simulink model "znn_we3"  (R2016b)
settings: Solver=VariableStepAuto  StartTime=0.0  StopTime=512  RelTol=1e-3  EnableMultiTasking=on
undefined symbols (not defined in the file): a, b
libraries: xbsIndex_r4 x143, simulink x3
settings Model: Creator=brad  LastModifiedBy=Brad Taylor
settings OptimizationCC: LifeSpan=inf
settings DebuggingCC: SFUnexpectedBacktrackingDiag=warning  SFNoUnconditionalDefaultTransitionDiag=warning  SFExecutionAtInitializationDiag=none
settings GRTTargetCC: TargetLangStandard=C89/C90 (ANSI)  GeneratePreprocessorConditionals=Disable all
settings ConfigComp: CovMetricSettings=dw  CovHtmlReporting=on  CovSaveCumulativeToWorkspaceVar=on  CovSaveSingleToWorkspaceVar=on  CovExternalEMLEnable=off

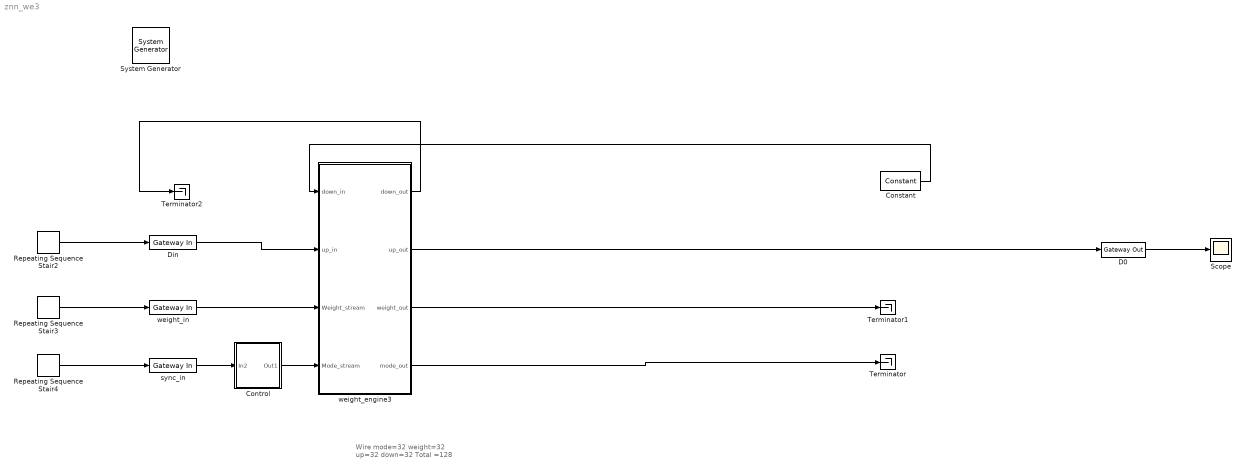
== system znn_we3 ==
  note: Wire
      | mode=32
      | weight=32
      | up=32
      | down=32
      | Total =128
  " System Generator" : xbsIndex_r4/ System Generator  Tag=genX  xilinxfamily=zynq  part=xc7z020  speed=-1  package=clg484  synthesis_tool=Vivado  clock_wrapper=Clock Enables  directory=D:/xsys/xwork/znn_we3  proj_type=Vivado  Synth_file=Vivado Synthesis Defaults  Impl_file=Vivado Implementation Defaults  testbench=off  simulink_period=1  sysclk_period=3.33  dcm_input_clock_period=10  incr_netlist=off  trim_vbits=Everywhere in SubSystem  dbl_ovrd=According to Block Masks  core_generation=According to Block Masks  run_coregen=off  deprecated_control=off  eval_field=0  block_type=sysgen
  Constant : xbsIndex_r4/Constant  const=1.0  gui_display_data_type=Fixed-point  arith_type=Unsigned  n_bits=36  bin_pt=0  preci_type=Single  exp_width=8  frac_width=24  explicit_period=on  period=1  equ=P=C  opselect=C  inp2=PCIN>>17  opr=+  inp1=P  carry=CIN  dbl_ovrd=off  block_type=constant
  Control : Subsystem
  D0 : xbsIndex_r4/Gateway Out  inherit_from_input=off  hdl_port=on  rows=1  columns=1  UseAsDAC=off  DACChannel='1'  interface=None  automatic_assignment=on  address_offset=hex2dec('00')  intf_name=''  intf_description=''  timing_constraint=None  locs_specified=off  LOCs={}  io_standard={}  block_type=gatewayout
  Din : xbsIndex_r4/Gateway In  gui_display_data_type=Fixed-point  arith_type=Unsigned  n_bits=36  bin_pt=0  preci_type=Single  exp_width=8  frac_width=24  rows=1  columns=1  quantization="Round  (unbiased: +/- Inf)"  overflow=Saturate  period=1  UseAsADC=off  ADCChannel='1'  interface=None  automatic_assignment=on  address_offset=hex2dec('00')  intf_name=''  intf_description=''  default_value=0  timing_constraint=None  locs_specified=off  LOCs={}  io_standard={}  inherit_from_input=off  hdl_port=on  dbl_ovrd=off  block_type=gatewayin
  Repeating Sequence Stair2 : simulink/Sources/Repeating Sequence Stair  OutValues=zeros(10,1)  tsamp=1  OutMin=[]  OutMax=[]  OutDataTypeStr=double  OutputDataTypeScalingMode=double  OutDataType=fixdt(0,8)  ConRadixGroup=Best Precision: Vector-wise  OutScaling=2^-12
  Repeating Sequence Stair3 : simulink/Sources/Repeating Sequence Stair  OutValues=1:10  tsamp=1  OutMin=[]  OutMax=[]  OutDataTypeStr=double  OutputDataTypeScalingMode=double  OutDataType=fixdt(0,8)  ConRadixGroup=Best Precision: Vector-wise  OutScaling=2^-12
  Repeating Sequence Stair4 : simulink/Sources/Repeating Sequence Stair  OutValues=[1, zeros(100,1)' ]  tsamp=1  OutMin=[]  OutMax=[]  OutDataTypeStr=double  OutputDataTypeScalingMode=double  OutDataType=fixdt(0,8)  ConRadixGroup=Best Precision: Vector-wise  OutScaling=2^-12
  Scope : Scope
  Terminator : Terminator
  Terminator1 : Terminator
  Terminator2 : Terminator
  sync_in : xbsIndex_r4/Gateway In  gui_display_data_type=Fixed-point  arith_type=Unsigned  n_bits=1  bin_pt=0  preci_type=Single  exp_width=8  frac_width=24  rows=1  columns=1  quantization="Round  (unbiased: +/- Inf)"  overflow=Saturate  period=1  UseAsADC=off  ADCChannel='1'  interface=None  automatic_assignment=on  address_offset=hex2dec('00')  intf_name=''  intf_description=''  default_value=0  timing_constraint=None  locs_specified=off  LOCs={}  io_standard={}  inherit_from_input=off  hdl_port=on  dbl_ovrd=off  block_type=gatewayin
  weight_engine3 : Subsystem
  weight_in : xbsIndex_r4/Gateway In  gui_display_data_type=Fixed-point  arith_type=Unsigned  n_bits=36  bin_pt=0  preci_type=Single  exp_width=8  frac_width=24  rows=1  columns=1  quantization="Round  (unbiased: +/- Inf)"  overflow=Saturate  period=1  UseAsADC=off  ADCChannel='1'  interface=None  automatic_assignment=on  address_offset=hex2dec('00')  intf_name=''  intf_description=''  default_value=0  timing_constraint=None  locs_specified=off  LOCs={}  io_standard={}  inherit_from_input=off  hdl_port=on  dbl_ovrd=off  block_type=gatewayin
  wires:
  D0/1 -> Scope/1
  Repeating Sequence Stair2/1 -> Din/1
  Repeating Sequence Stair3/1 -> weight_in/1
  Repeating Sequence Stair4/1 -> sync_in/1
  weight_engine3/3(weight_out) -> Terminator1/1
  weight_engine3/4(mode_out) -> Terminator/1
  Control/1(Out1) -> weight_engine3/4(Mode_stream)
  weight_in/1 -> weight_engine3/3(Weight_stream)
  sync_in/1 -> Control/1(In2)
  weight_engine3/2(up_out) -> D0/1
  Din/1 -> weight_engine3/2(up_in)
  weight_engine3/1(down_out) -> Terminator2/1
  Constant/1 -> weight_engine3/1(down_in)

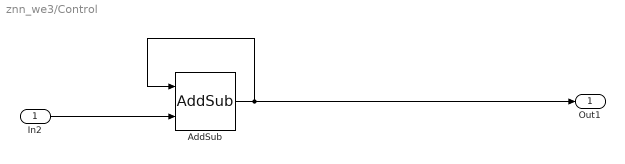
== system znn_we3/Control ==
  In2 : Inport
  AddSub : xbsIndex_r4/AddSub  mode=Addition  use_carryin=off  use_carryout=off  en=off  latency=1  precision=User Defined  arith_type=Unsigned  n_bits=36  bin_pt=0  quantization=Truncate  overflow=Wrap  use_behavioral_HDL=off  hw_selection=Fabric  pipelined=off  dbl_ovrd=off  block_type=addsub
  Out1 : Outport
  wires:
  In2/1 -> AddSub/2
  AddSub/1 -> AddSub/1, Out1/1

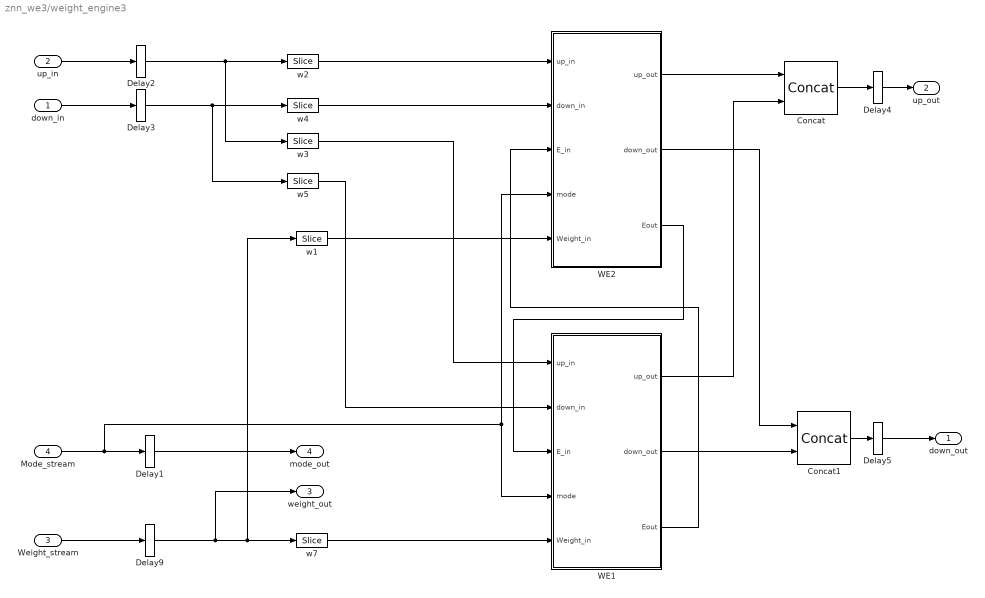
== system znn_we3/weight_engine3 ==
  down_in : Inport
  up_in : Inport  Port=2
  Weight_stream : Inport  Port=3
  Mode_stream : Inport  Port=4
  Concat : xbsIndex_r4/Concat  num_inputs=2  dbl_ovrd=off  block_type=concat
  Concat1 : xbsIndex_r4/Concat  num_inputs=2  dbl_ovrd=off  block_type=concat
  Delay{1..5,9} (6 alike) : xbsIndex_r4/Delay  rst=off  infoeditControl=Selection of Reset will increase slice count due to use of real FFs and instead of SRLs  en=off  latency=1  reg_retiming=off  dbl_ovrd=off  block_type=delay
      settings: infoedit=Hardware notes: A delay line is a chain, each link of which is an SRL16 or SRL32 followed by a flip-flop.
  WE1 : Subsystem
  WE2 : Subsystem
  w1 : xbsIndex_r4/Slice  nbits=1  boolean_output=off  mode=Two Bit Locations  bit1=35  base1=LSB of Input  bit0=18  base0=LSB of Input  dbl_ovrd=off  block_type=slice
  w2 : xbsIndex_r4/Slice  nbits=1  boolean_output=off  mode=Two Bit Locations  bit1=35  base1=LSB of Input  bit0=18  base0=LSB of Input  dbl_ovrd=off  block_type=slice
  w3 : xbsIndex_r4/Slice  nbits=1  boolean_output=off  mode=Two Bit Locations  bit1=17  base1=LSB of Input  bit0=0  base0=LSB of Input  dbl_ovrd=off  block_type=slice
  w4 : xbsIndex_r4/Slice  nbits=1  boolean_output=off  mode=Two Bit Locations  bit1=35  base1=LSB of Input  bit0=18  base0=LSB of Input  dbl_ovrd=off  block_type=slice
  w5 : xbsIndex_r4/Slice  nbits=1  boolean_output=off  mode=Two Bit Locations  bit1=17  base1=LSB of Input  bit0=0  base0=LSB of Input  dbl_ovrd=off  block_type=slice
  w7 : xbsIndex_r4/Slice  nbits=1  boolean_output=off  mode=Two Bit Locations  bit1=17  base1=LSB of Input  bit0=0  base0=LSB of Input  dbl_ovrd=off  block_type=slice
  down_out : Outport
  up_out : Outport  Port=2
  weight_out : Outport  Port=3
  mode_out : Outport  Port=4
  wires:
  Weight_stream/1 -> Delay9/1
  Delay9/1 -> weight_out/1, w7/1, w1/1
  WE2/2(down_out) -> Concat1/1
  down_in/1 -> Delay3/1
  Mode_stream/1 -> Delay1/1, WE2/4(mode), WE1/4(mode)
  WE1/2(down_out) -> Concat1/2
  WE1/1(up_out) -> Concat/2
  WE1/3(Eout) -> WE2/3(E_in)
  WE2/3(Eout) -> WE1/3(E_in)
  w7/1 -> WE1/5(Weight_in)
  w1/1 -> WE2/5(Weight_in)
  Concat/1 -> Delay4/1
  Concat1/1 -> Delay5/1
  w2/1 -> WE2/1(up_in)
  up_in/1 -> Delay2/1
  w3/1 -> WE1/1(up_in)
  w4/1 -> WE2/2(down_in)
  w5/1 -> WE1/2(down_in)
  Delay1/1 -> mode_out/1
  Delay2/1 -> w3/1, w2/1
  Delay3/1 -> w5/1, w4/1
  Delay4/1 -> up_out/1
  Delay5/1 -> down_out/1
  WE2/1(up_out) -> Concat/1

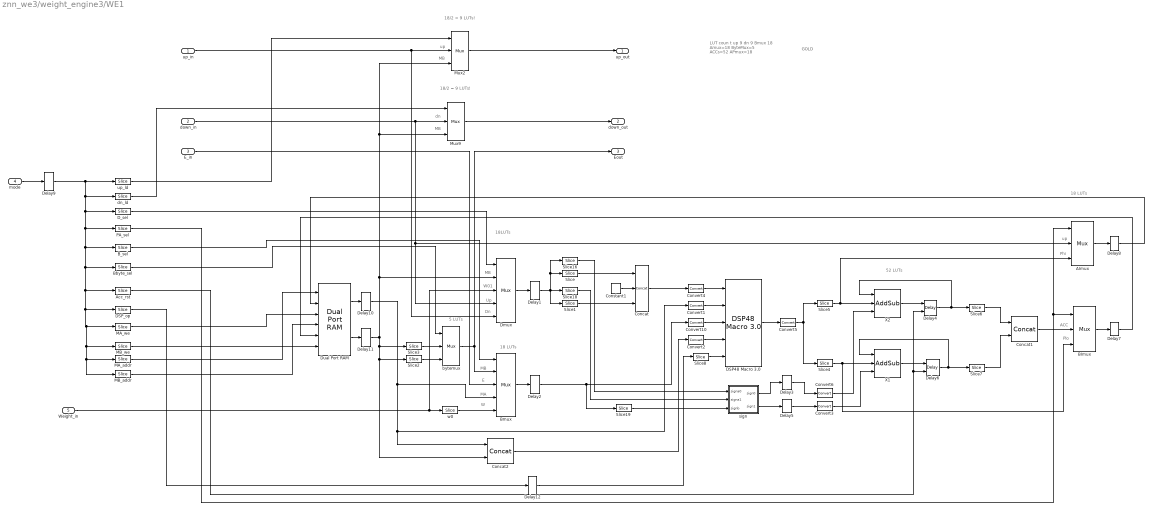
== system znn_we3/weight_engine3/WE1 ==
  note: Plo
  note: ACC
  note: Phi
  note: up
  note: MB
  note: dn
  note: MB
  note: up
  note: 5 LUTs
  note: Dn
  note: Up
  note: W01
  note: MB
  note: W
  note: E
  note: GOLD
  note: LUT coun t
      | up 9
      | dn 9
      | Bmux 18
      | Amux=18
      | ByteMux=5
      | ACCs=52
      | APmux=18
  note: 18 LUTs
  note: 18LUTs
  note: 18 LUTs
  note: 52 LUTs
  note: MA
  note: MB
  note: 18/2 = 9 LUTs!
  note: 18/2 = 9 LUTs!
  up_in : Inport
  down_in : Inport  Port=2
  E_in : Inport  Port=3
  mode : Inport  Port=4
  Weight_in : Inport  Port=5
  AImux : xbsIndex_r4/Mux  inputs=2  en=off  latency=0  precision=Full  arith_type=Unsigned  n_bits=16  bin_pt=14  quantization=Truncate  overflow=Wrap  dbl_ovrd=off  block_type=mux
  Acc_rst : xbsIndex_r4/Slice  nbits=1  boolean_output=on  mode=Two Bit Locations  bit1=26  base1=LSB of Input  bit0=26  base0=LSB of Input  dbl_ovrd=off  block_type=slice
  BImux : xbsIndex_r4/Mux  inputs=2  en=off  latency=0  precision=Full  arith_type=Unsigned  n_bits=16  bin_pt=14  quantization=Truncate  overflow=Wrap  dbl_ovrd=off  block_type=mux
  B_sel : xbsIndex_r4/Slice  nbits=1  boolean_output=off  mode=Two Bit Locations  bit1=29  base1=LSB of Input  bit0=28  base0=LSB of Input  dbl_ovrd=off  block_type=slice
  Bbyte_sel : xbsIndex_r4/Slice  nbits=1  boolean_output=off  mode=Two Bit Locations  bit1=27  base1=LSB of Input  bit0=27  base0=LSB of Input  dbl_ovrd=off  block_type=slice
  Bmux : xbsIndex_r4/Mux  inputs=4  en=off  latency=0  precision=Full  arith_type=Unsigned  n_bits=16  bin_pt=14  quantization=Truncate  overflow=Wrap  dbl_ovrd=off  block_type=mux
  Concat : xbsIndex_r4/Concat  num_inputs=3  dbl_ovrd=off  block_type=concat
  Concat1 : xbsIndex_r4/Concat  num_inputs=2  dbl_ovrd=off  block_type=concat
  Concat2 : xbsIndex_r4/Concat  num_inputs=2  dbl_ovrd=off  block_type=concat
  Constant1 : xbsIndex_r4/Constant  const=0  gui_display_data_type=Fixed-point  arith_type=Unsigned  n_bits=8  bin_pt=0  preci_type=Single  exp_width=8  frac_width=24  explicit_period=off  period=1  equ=P=C  opselect=C  inp2=PCIN>>17  opr=+  inp1=P  carry=CIN  dbl_ovrd=off  block_type=constant
  Convert1 : xbsIndex_r4/Convert  gui_display_data_type=Fixed-point  arith_type="Signed  (2's comp)"  n_bits=18  bin_pt=0  float_type=Single  exp_bits=8  fraction_bits=24  quantization=Truncate  overflow=Wrap  en=off  latency=0  pipeline=off  dbl_ovrd=off  block_type=convert
  Convert10 : xbsIndex_r4/Convert  gui_display_data_type=Fixed-point  arith_type="Signed  (2's comp)"  n_bits=18  bin_pt=0  float_type=Single  exp_bits=8  fraction_bits=24  quantization=Truncate  overflow=Wrap  en=off  latency=0  pipeline=off  dbl_ovrd=off  block_type=convert
  Convert2 : xbsIndex_r4/Convert  gui_display_data_type=Fixed-point  arith_type="Signed  (2's comp)"  n_bits=36  bin_pt=0  float_type=Single  exp_bits=8  fraction_bits=24  quantization=Truncate  overflow=Wrap  en=off  latency=0  pipeline=off  dbl_ovrd=off  block_type=convert
  Convert3 : xbsIndex_r4/Convert  gui_display_data_type=Boolean  arith_type=Boolean  n_bits=9  bin_pt=0  float_type=Single  exp_bits=8  fraction_bits=24  quantization=Truncate  overflow=Wrap  en=off  latency=0  pipeline=off  dbl_ovrd=off  block_type=convert
  Convert4 : xbsIndex_r4/Convert  gui_display_data_type=Fixed-point  arith_type="Signed  (2's comp)"  n_bits=23  bin_pt=0  float_type=Single  exp_bits=8  fraction_bits=24  quantization=Truncate  overflow=Wrap  en=off  latency=0  pipeline=off  dbl_ovrd=off  block_type=convert
  Convert5 : xbsIndex_r4/Convert  gui_display_data_type=Fixed-point  arith_type=Unsigned  n_bits=48  bin_pt=0  float_type=Single  exp_bits=8  fraction_bits=24  quantization=Truncate  overflow=Wrap  en=off  latency=0  pipeline=off  dbl_ovrd=off  block_type=convert
  Convert6 : xbsIndex_r4/Convert  gui_display_data_type=Boolean  arith_type=Boolean  n_bits=9  bin_pt=0  float_type=Single  exp_bits=8  fraction_bits=24  quantization=Truncate  overflow=Wrap  en=off  latency=0  pipeline=off  dbl_ovrd=off  block_type=convert
  "DSP48 Macro 3.0 " : xbsIndex_r4/DSP48 Macro 3.0   dsptype=Target XtremeDSP Slice: DSP48E1  instruction_list=|  show_filtered=on  pipeline_options=By_Tier  dspimage=?  tier_1=off  tier_2=off  tier_3=off  tier_4=on  tier_5=on  tier_6=on  dreg_1=off  dreg_2=off  dreg_3=off  areg_1=off  areg_2=off  areg_3=off  areg_4=on  breg_1=off  breg_2=off  breg_3=off  breg_4=on  mreg_5=on  concatreg_3=off  concatreg_4=off  concatreg_5=off  creg_1=off  creg_2=off  creg_3=off  creg_4=on  creg_5=on  preg_6=on  cinreg_1=off  cinreg_2=off  cinreg_3=off  cinreg_4=off  cinreg_5=off  opreg_1=off  opreg_2=off  opreg_3=off  opreg_4=on  opreg_5=on  output_properties=Full_Precision  p_width=48  p_binarywidth=0  has_acout=off  has_bcout=off  has_pcout=off  has_carryout=off  has_carrycascout=off  has_ce=off  has_d_ce=off  has_a_ce=off  has_b_ce=off  has_concat_ce=off  has_c_ce=off  has_m_ce=off  has_p_ce=off  has_sel_ce=off  has_sclr=off  has_d_sclr=off  has_a_sclr=off  has_b_sclr=off  has_concat_sclr=off  has_c_sclr=off  has_m_sclr=off  has_p_sclr=off  has_sel_sclr=off  use_dsp48=on  simulation_type=fast_sim  simulation_model=sysgen:xbip_dsp48_macro_v3_0  gui_behaviour=Sysgen  instruction1='#'  ip_name=DSP48 Macro  ip_version=3.0  dsptool_ready=true  ipcore_usecache=true  ipcore_useipmodelcache=true  wrapper_available=true  port_translation_map={ 'ce' => 'en', 'sclr' => 'rst'}  ipcore_latency_function='has_combinational'  structural_sim=false  ipcore_verbose=false  ipcore_port_config={ 'carryin' => { 'arith' => 'ufix', 'binpt' => 0.00000000000, 'width' => 1.00000000000}, 'carrycascin' => { 'arith' => 'ufix', 'binpt' => 0.00000000000, 'width' => 1.00000000000}, 'carrycascout' => { 'arith' => 'ufix', 'binpt' => 0.00000000000, 'width' => 1.00000000000}, 'carryout' => { 'arith' => 'ufix', 'binpt' => 0.00000000000, 'width' => 1.00000000000}}  ipcore_xco_need_fpga_part=true  block_type=xbip_dsp48_macro_v3_0
      | A*B
      | D*B
      | C
      settings: infoedit=<html>Valid operands: CONCAT, P, C, PCIN, P>>17, PCIN>>17, CARRYIN, CARRYCASCIN, ACIN, A, BCIN,B<br><br>Valid operators: +, -, *, ()<br><br>Valid functions: RNDSIMPLE, RNDSYM<br><br>Instructions are case insensitive and tolerate spaces.</html>
  DSP_op : xbsIndex_r4/Slice  nbits=1  boolean_output=off  mode=Two Bit Locations  bit1=25  base1=LSB of Input  bit0=22  base0=LSB of Input  dbl_ovrd=off  block_type=slice
  D_sel : xbsIndex_r4/Slice  nbits=1  boolean_output=off  mode=Two Bit Locations  bit1=32  base1=LSB of Input  bit0=31  base0=LSB of Input  dbl_ovrd=off  block_type=slice
  Delay{1..2,7..12} (8 alike) : xbsIndex_r4/Delay  rst=off  infoeditControl=Selection of Reset will increase slice count due to use of real FFs and instead of SRLs  en=off  latency=1  reg_retiming=off  dbl_ovrd=off  block_type=delay
  Delay3 : xbsIndex_r4/Delay  rst=off  infoeditControl=Selection of Reset will increase slice count due to use of real FFs and instead of SRLs  en=off  latency=3  reg_retiming=off  dbl_ovrd=off  block_type=delay
  Delay4 : xbsIndex_r4/Delay  rst=on  infoeditControl=Selection of Reset will increase slice count due to use of real FFs and instead of SRLs  en=off  latency=1  reg_retiming=off  dbl_ovrd=off  block_type=delay
  Delay5 : xbsIndex_r4/Delay  rst=off  infoeditControl=Selection of Reset will increase slice count due to use of real FFs and instead of SRLs  en=off  latency=3  reg_retiming=off  dbl_ovrd=off  block_type=delay
  Delay6 : xbsIndex_r4/Delay  rst=on  infoeditControl=Selection of Reset will increase slice count due to use of real FFs and instead of SRLs  en=off  latency=1  reg_retiming=off  dbl_ovrd=off  block_type=delay
  Dmux : xbsIndex_r4/Mux  inputs=4  en=off  latency=0  precision=Full  arith_type=Unsigned  n_bits=16  bin_pt=14  quantization=Truncate  overflow=Wrap  dbl_ovrd=off  block_type=mux
  Dual Port RAM : xbsIndex_r4/Dual Port RAM  depth=1024  initVector=1:100  distributed_mem=Block RAM  init_a=0  init_b=0  rst_a=off  rst_b=off  en_a=off  en_b=off  latency=2  write_mode_A=Read After Write  write_mode_B=Read After Write  optimize=Speed  dbl_ovrd=off  block_type=dpram
  MA_addr : xbsIndex_r4/Slice  nbits=1  boolean_output=off  mode=Two Bit Locations  bit1=19  base1=LSB of Input  bit0=10  base0=LSB of Input  dbl_ovrd=off  block_type=slice
  MA_we : xbsIndex_r4/Slice  nbits=1  boolean_output=on  mode=Two Bit Locations  bit1=21  base1=LSB of Input  bit0=21  base0=LSB of Input  dbl_ovrd=off  block_type=slice
  MB_addr : xbsIndex_r4/Slice  nbits=1  boolean_output=off  mode=Two Bit Locations  bit1=9  base1=LSB of Input  bit0=0  base0=LSB of Input  dbl_ovrd=off  block_type=slice
  MB_we : xbsIndex_r4/Slice  nbits=1  boolean_output=on  mode=Two Bit Locations  bit1=20  base1=LSB of Input  bit0=20  base0=LSB of Input  dbl_ovrd=off  block_type=slice
  Mux2 : xbsIndex_r4/Mux  inputs=2  en=off  latency=0  precision=Full  arith_type=Unsigned  n_bits=16  bin_pt=14  quantization=Truncate  overflow=Wrap  dbl_ovrd=off  block_type=mux
  Mux9 : xbsIndex_r4/Mux  inputs=2  en=off  latency=0  precision=Full  arith_type=Unsigned  n_bits=16  bin_pt=14  quantization=Truncate  overflow=Wrap  dbl_ovrd=off  block_type=mux
  PA_sel : xbsIndex_r4/Slice  nbits=1  boolean_output=off  mode=Two Bit Locations  bit1=30  base1=LSB of Input  bit0=30  base0=LSB of Input  dbl_ovrd=off  block_type=slice
  Slice : xbsIndex_r4/Slice  nbits=1  boolean_output=off  mode=Two Bit Locations  bit1=16  base1=LSB of Input  bit0=9  base0=LSB of Input  dbl_ovrd=off  block_type=slice
  Slice1 : xbsIndex_r4/Slice  nbits=1  boolean_output=off  mode=Two Bit Locations  bit1=7  base1=LSB of Input  bit0=0  base0=LSB of Input  dbl_ovrd=off  block_type=slice
  Slice16 : xbsIndex_r4/Slice  nbits=1  boolean_output=off  mode=Two Bit Locations  bit1=16  base1=LSB of Input  bit0=16  base0=LSB of Input  dbl_ovrd=off  block_type=slice
  Slice18 : xbsIndex_r4/Slice  nbits=1  boolean_output=off  mode=Two Bit Locations  bit1=8  base1=LSB of Input  bit0=8  base0=LSB of Input  dbl_ovrd=off  block_type=slice
  Slice19 : xbsIndex_r4/Slice  nbits=1  boolean_output=off  mode=Two Bit Locations  bit1=8  base1=LSB of Input  bit0=8  base0=LSB of Input  dbl_ovrd=off  block_type=slice
  Slice2 : xbsIndex_r4/Slice  nbits=1  boolean_output=off  mode=Two Bit Locations  bit1=17  base1=LSB of Input  bit0=9  base0=LSB of Input  dbl_ovrd=off  block_type=slice
  Slice3 : xbsIndex_r4/Slice  nbits=1  boolean_output=off  mode=Two Bit Locations  bit1=8  base1=LSB of Input  bit0=0  base0=LSB of Input  dbl_ovrd=off  block_type=slice
  Slice4 : xbsIndex_r4/Slice  nbits=1  boolean_output=off  mode=Two Bit Locations  bit1=17  base1=LSB of Input  bit0=0  base0=LSB of Input  dbl_ovrd=off  block_type=slice
  Slice5 : xbsIndex_r4/Slice  nbits=1  boolean_output=off  mode=Two Bit Locations  bit1=35  base1=LSB of Input  bit0=18  base0=LSB of Input  dbl_ovrd=off  block_type=slice
  Slice6 : xbsIndex_r4/Slice  nbits=1  boolean_output=off  mode=Two Bit Locations  bit1=24  base1=LSB of Input  bit0=17  base0=LSB of Input  dbl_ovrd=off  block_type=slice
  Slice7 : xbsIndex_r4/Slice  nbits=1  boolean_output=off  mode=Two Bit Locations  bit1=24  base1=LSB of Input  bit0=17  base0=LSB of Input  dbl_ovrd=off  block_type=slice
  Slice8 : xbsIndex_r4/Slice  nbits=1  boolean_output=off  mode=Two Bit Locations  bit1=1  base1=LSB of Input  bit0=0  base0=LSB of Input  dbl_ovrd=off  block_type=slice
  X1 : xbsIndex_r4/AddSub  mode=Addition or Subtraction  use_carryin=off  use_carryout=off  en=off  latency=0  precision=User Defined  arith_type="Signed  (2's comp)"  n_bits=26  bin_pt=0  quantization=Truncate  overflow=Wrap  use_behavioral_HDL=off  hw_selection=Fabric  pipelined=off  dbl_ovrd=off  block_type=addsub
  X2 : xbsIndex_r4/AddSub  mode=Addition or Subtraction  use_carryin=off  use_carryout=off  en=off  latency=0  precision=User Defined  arith_type="Signed  (2's comp)"  n_bits=26  bin_pt=0  quantization=Truncate  overflow=Wrap  use_behavioral_HDL=off  hw_selection=Fabric  pipelined=off  dbl_ovrd=off  block_type=addsub
  bytemux : xbsIndex_r4/Mux  inputs=2  en=off  latency=0  precision=Full  arith_type=Unsigned  n_bits=16  bin_pt=14  quantization=Truncate  overflow=Wrap  dbl_ovrd=off  block_type=mux
  dn_ld : xbsIndex_r4/Slice  nbits=1  boolean_output=off  mode=Two Bit Locations  bit1=33  base1=LSB of Input  bit0=33  base0=LSB of Input  dbl_ovrd=off  block_type=slice
  sign : Subsystem
  up_ld : xbsIndex_r4/Slice  nbits=1  boolean_output=off  mode=Two Bit Locations  bit1=34  base1=LSB of Input  bit0=34  base0=LSB of Input  dbl_ovrd=off  block_type=slice
  w0 : xbsIndex_r4/Slice  nbits=1  boolean_output=off  mode=Two Bit Locations  bit1=8  base1=LSB of Input  bit0=0  base0=LSB of Input  dbl_ovrd=off  block_type=slice
  up_out : Outport
  down_out : Outport  Port=2
  Eout : Outport  Port=3
  wires:
  Convert4/1 -> "DSP48 Macro 3.0 "/1
  sign/2(sign1) -> Delay5/1
  w0/1 -> Bmux/5
  Convert10/1 -> "DSP48 Macro 3.0 "/3
  Dmux/1 -> Delay1/1
  Convert1/1 -> "DSP48 Macro 3.0 "/2
  Dual Port RAM/1 -> Delay10/1
  Slice2/1 -> bytemux/3
  Slice18/1 -> sign/2(signa1)
  Slice19/1 -> sign/3(signb)
  sign/1(sign0) -> Delay3/1
  PA_sel/1 -> BImux/1, AImux/1
  B_sel/1 -> Bmux/1
  Bbyte_sel/1 -> bytemux/1
  X1/1 -> Delay6/1
  MA_addr/1 -> Dual Port RAM/1
  MA_we/1 -> Dual Port RAM/3
  Slice5/1 -> AImux/3, X2/2
  Concat1/1 -> BImux/2
  Delay6/1 -> Slice7/1, X1/1
  Convert5/1 -> Slice5/1, Slice4/1
  X2/1 -> Delay4/1
  Acc_rst/1 -> Delay4/2, Delay6/2
  Delay4/1 -> Slice6/1, X2/1
  Slice4/1 -> BImux/3, X1/2
  Convert3/1 -> X1/3
  Constant1/1 -> Concat/2
  Slice6/1 -> Concat1/1
  "DSP48 Macro 3.0 "/1 -> Convert5/1
  Slice7/1 -> Concat1/2
  BImux/1 -> Delay7/1
  MB_we/1 -> Dual Port RAM/6
  Slice1/1 -> Concat/3
  Slice/1 -> Concat/1
  Slice3/1 -> bytemux/2
  Bmux/1 -> Delay2/1
  bytemux/1 -> Eout/1, Bmux/2
  Dual Port RAM/2 -> Delay11/1
  Weight_in/1 -> Dmux/3, w0/1
  Slice16/1 -> sign/1(signa0)
  Mux9/1 -> down_out/1
  dn_ld/1 -> Mux9/1
  D_sel/1 -> Dmux/1
  down_in/1 -> AImux/2, Dmux/4, Mux9/2
  Concat2/1 -> Convert2/1
  mode/1 -> Delay9/1
  up_in/1 -> Mux2/2, Dmux/5
  MB_addr/1 -> Dual Port RAM/4
  E_in/1 -> Bmux/3
  up_ld/1 -> Mux2/1
  Convert2/1 -> "DSP48 Macro 3.0 "/4
  Convert6/1 -> X2/3
  AImux/1 -> Delay8/1
  Mux2/1 -> up_out/1
  Delay1/1 -> Slice1/1, Slice18/1, Slice/1, Slice16/1
  Delay2/1 -> Slice19/1, Convert10/1
  Delay3/1 -> Convert6/1
  Delay5/1 -> Convert3/1
  Delay7/1 -> Dual Port RAM/5
  Delay8/1 -> Dual Port RAM/2
  Concat/1 -> Convert4/1
  Slice8/1 -> "DSP48 Macro 3.0 "/5
  DSP_op/1 -> Delay12/1
  Delay9/1 -> dn_ld/1, PA_sel/1, B_sel/1, MB_addr/1, MA_addr/1, MB_we/1, MA_we/1, DSP_op/1, Acc_rst/1, Bbyte_sel/1, D_sel/1, up_ld/1
  Delay10/1 -> Bmux/4, Convert1/1, Concat2/1
  Delay11/1 -> Slice3/1, Slice2/1, Concat2/2, Mux2/3, Mux9/3, Dmux/2
  Delay12/1 -> Slice8/1

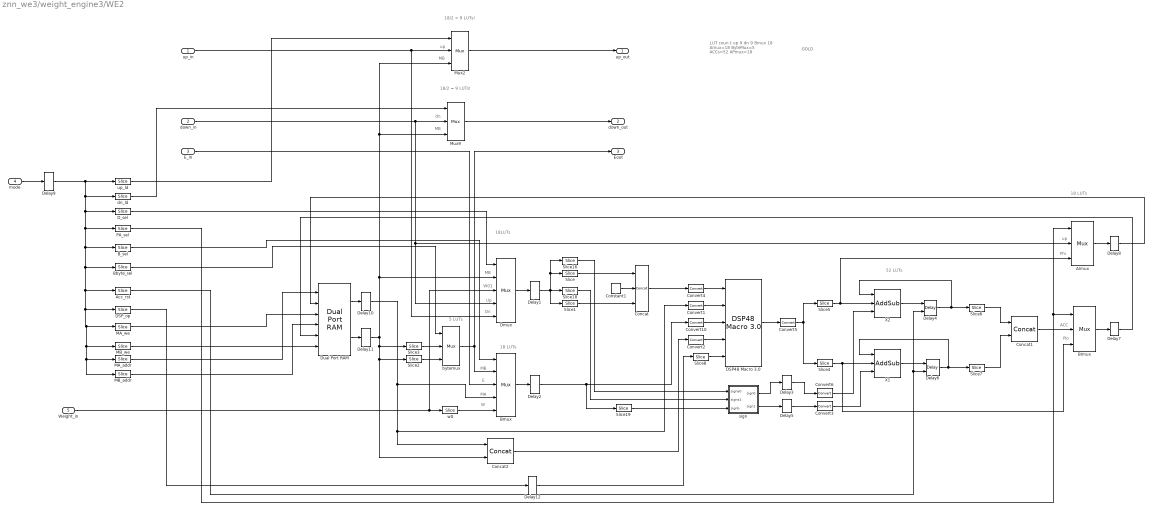
== system znn_we3/weight_engine3/WE2 ==
  note: Plo
  note: ACC
  note: Phi
  note: up
  note: MB
  note: dn
  note: MB
  note: up
  note: 5 LUTs
  note: Dn
  note: Up
  note: W01
  note: MB
  note: W
  note: E
  note: GOLD
  note: LUT coun t
      | up 9
      | dn 9
      | Bmux 18
      | Amux=18
      | ByteMux=5
      | ACCs=52
      | APmux=18
  note: 18 LUTs
  note: 18LUTs
  note: 18 LUTs
  note: 52 LUTs
  note: MA
  note: MB
  note: 18/2 = 9 LUTs!
  note: 18/2 = 9 LUTs!
  up_in : Inport
  down_in : Inport  Port=2
  E_in : Inport  Port=3
  mode : Inport  Port=4
  Weight_in : Inport  Port=5
  AImux : xbsIndex_r4/Mux  inputs=2  en=off  latency=0  precision=Full  arith_type=Unsigned  n_bits=16  bin_pt=14  quantization=Truncate  overflow=Wrap  dbl_ovrd=off  block_type=mux
  Acc_rst : xbsIndex_r4/Slice  nbits=1  boolean_output=on  mode=Two Bit Locations  bit1=26  base1=LSB of Input  bit0=26  base0=LSB of Input  dbl_ovrd=off  block_type=slice
  BImux : xbsIndex_r4/Mux  inputs=2  en=off  latency=0  precision=Full  arith_type=Unsigned  n_bits=16  bin_pt=14  quantization=Truncate  overflow=Wrap  dbl_ovrd=off  block_type=mux
  B_sel : xbsIndex_r4/Slice  nbits=1  boolean_output=off  mode=Two Bit Locations  bit1=29  base1=LSB of Input  bit0=28  base0=LSB of Input  dbl_ovrd=off  block_type=slice
  Bbyte_sel : xbsIndex_r4/Slice  nbits=1  boolean_output=off  mode=Two Bit Locations  bit1=27  base1=LSB of Input  bit0=27  base0=LSB of Input  dbl_ovrd=off  block_type=slice
  Bmux : xbsIndex_r4/Mux  inputs=4  en=off  latency=0  precision=Full  arith_type=Unsigned  n_bits=16  bin_pt=14  quantization=Truncate  overflow=Wrap  dbl_ovrd=off  block_type=mux
  Concat : xbsIndex_r4/Concat  num_inputs=3  dbl_ovrd=off  block_type=concat
  Concat1 : xbsIndex_r4/Concat  num_inputs=2  dbl_ovrd=off  block_type=concat
  Concat2 : xbsIndex_r4/Concat  num_inputs=2  dbl_ovrd=off  block_type=concat
  Constant1 : xbsIndex_r4/Constant  const=0  gui_display_data_type=Fixed-point  arith_type=Unsigned  n_bits=8  bin_pt=0  preci_type=Single  exp_width=8  frac_width=24  explicit_period=off  period=1  equ=P=C  opselect=C  inp2=PCIN>>17  opr=+  inp1=P  carry=CIN  dbl_ovrd=off  block_type=constant
  Convert1 : xbsIndex_r4/Convert  gui_display_data_type=Fixed-point  arith_type="Signed  (2's comp)"  n_bits=18  bin_pt=0  float_type=Single  exp_bits=8  fraction_bits=24  quantization=Truncate  overflow=Wrap  en=off  latency=0  pipeline=off  dbl_ovrd=off  block_type=convert
  Convert10 : xbsIndex_r4/Convert  gui_display_data_type=Fixed-point  arith_type="Signed  (2's comp)"  n_bits=18  bin_pt=0  float_type=Single  exp_bits=8  fraction_bits=24  quantization=Truncate  overflow=Wrap  en=off  latency=0  pipeline=off  dbl_ovrd=off  block_type=convert
  Convert2 : xbsIndex_r4/Convert  gui_display_data_type=Fixed-point  arith_type="Signed  (2's comp)"  n_bits=36  bin_pt=0  float_type=Single  exp_bits=8  fraction_bits=24  quantization=Truncate  overflow=Wrap  en=off  latency=0  pipeline=off  dbl_ovrd=off  block_type=convert
  Convert3 : xbsIndex_r4/Convert  gui_display_data_type=Boolean  arith_type=Boolean  n_bits=9  bin_pt=0  float_type=Single  exp_bits=8  fraction_bits=24  quantization=Truncate  overflow=Wrap  en=off  latency=0  pipeline=off  dbl_ovrd=off  block_type=convert
  Convert4 : xbsIndex_r4/Convert  gui_display_data_type=Fixed-point  arith_type="Signed  (2's comp)"  n_bits=23  bin_pt=0  float_type=Single  exp_bits=8  fraction_bits=24  quantization=Truncate  overflow=Wrap  en=off  latency=0  pipeline=off  dbl_ovrd=off  block_type=convert
  Convert5 : xbsIndex_r4/Convert  gui_display_data_type=Fixed-point  arith_type=Unsigned  n_bits=48  bin_pt=0  float_type=Single  exp_bits=8  fraction_bits=24  quantization=Truncate  overflow=Wrap  en=off  latency=0  pipeline=off  dbl_ovrd=off  block_type=convert
  Convert6 : xbsIndex_r4/Convert  gui_display_data_type=Boolean  arith_type=Boolean  n_bits=9  bin_pt=0  float_type=Single  exp_bits=8  fraction_bits=24  quantization=Truncate  overflow=Wrap  en=off  latency=0  pipeline=off  dbl_ovrd=off  block_type=convert
  "DSP48 Macro 3.0 " : xbsIndex_r4/DSP48 Macro 3.0   dsptype=Target XtremeDSP Slice: DSP48E1  instruction_list=|  show_filtered=on  pipeline_options=By_Tier  dspimage=?  tier_1=off  tier_2=off  tier_3=off  tier_4=on  tier_5=on  tier_6=on  dreg_1=off  dreg_2=off  dreg_3=off  areg_1=off  areg_2=off  areg_3=off  areg_4=on  breg_1=off  breg_2=off  breg_3=off  breg_4=on  mreg_5=on  concatreg_3=off  concatreg_4=off  concatreg_5=off  creg_1=off  creg_2=off  creg_3=off  creg_4=on  creg_5=on  preg_6=on  cinreg_1=off  cinreg_2=off  cinreg_3=off  cinreg_4=off  cinreg_5=off  opreg_1=off  opreg_2=off  opreg_3=off  opreg_4=on  opreg_5=on  output_properties=Full_Precision  p_width=48  p_binarywidth=0  has_acout=off  has_bcout=off  has_pcout=off  has_carryout=off  has_carrycascout=off  has_ce=off  has_d_ce=off  has_a_ce=off  has_b_ce=off  has_concat_ce=off  has_c_ce=off  has_m_ce=off  has_p_ce=off  has_sel_ce=off  has_sclr=off  has_d_sclr=off  has_a_sclr=off  has_b_sclr=off  has_concat_sclr=off  has_c_sclr=off  has_m_sclr=off  has_p_sclr=off  has_sel_sclr=off  use_dsp48=on  simulation_type=fast_sim  simulation_model=sysgen:xbip_dsp48_macro_v3_0  gui_behaviour=Sysgen  instruction1='#'  ip_name=DSP48 Macro  ip_version=3.0  dsptool_ready=true  ipcore_usecache=true  ipcore_useipmodelcache=true  wrapper_available=true  port_translation_map={ 'ce' => 'en', 'sclr' => 'rst'}  ipcore_latency_function='has_combinational'  structural_sim=false  ipcore_verbose=false  ipcore_port_config={ 'carryin' => { 'arith' => 'ufix', 'binpt' => 0.00000000000, 'width' => 1.00000000000}, 'carrycascin' => { 'arith' => 'ufix', 'binpt' => 0.00000000000, 'width' => 1.00000000000}, 'carrycascout' => { 'arith' => 'ufix', 'binpt' => 0.00000000000, 'width' => 1.00000000000}, 'carryout' => { 'arith' => 'ufix', 'binpt' => 0.00000000000, 'width' => 1.00000000000}}  ipcore_xco_need_fpga_part=true  block_type=xbip_dsp48_macro_v3_0
      | A*B
      | D*B
      | C
      settings: infoedit=<html>Valid operands: CONCAT, P, C, PCIN, P>>17, PCIN>>17, CARRYIN, CARRYCASCIN, ACIN, A, BCIN,B<br><br>Valid operators: +, -, *, ()<br><br>Valid functions: RNDSIMPLE, RNDSYM<br><br>Instructions are case insensitive and tolerate spaces.</html>
  DSP_op : xbsIndex_r4/Slice  nbits=1  boolean_output=off  mode=Two Bit Locations  bit1=25  base1=LSB of Input  bit0=22  base0=LSB of Input  dbl_ovrd=off  block_type=slice
  D_sel : xbsIndex_r4/Slice  nbits=1  boolean_output=off  mode=Two Bit Locations  bit1=32  base1=LSB of Input  bit0=31  base0=LSB of Input  dbl_ovrd=off  block_type=slice
  Delay{1..2,7..12} (8 alike) : xbsIndex_r4/Delay  rst=off  infoeditControl=Selection of Reset will increase slice count due to use of real FFs and instead of SRLs  en=off  latency=1  reg_retiming=off  dbl_ovrd=off  block_type=delay
  Delay3 : xbsIndex_r4/Delay  rst=off  infoeditControl=Selection of Reset will increase slice count due to use of real FFs and instead of SRLs  en=off  latency=3  reg_retiming=off  dbl_ovrd=off  block_type=delay
  Delay4 : xbsIndex_r4/Delay  rst=on  infoeditControl=Selection of Reset will increase slice count due to use of real FFs and instead of SRLs  en=off  latency=1  reg_retiming=off  dbl_ovrd=off  block_type=delay
  Delay5 : xbsIndex_r4/Delay  rst=off  infoeditControl=Selection of Reset will increase slice count due to use of real FFs and instead of SRLs  en=off  latency=3  reg_retiming=off  dbl_ovrd=off  block_type=delay
  Delay6 : xbsIndex_r4/Delay  rst=on  infoeditControl=Selection of Reset will increase slice count due to use of real FFs and instead of SRLs  en=off  latency=1  reg_retiming=off  dbl_ovrd=off  block_type=delay
  Dmux : xbsIndex_r4/Mux  inputs=4  en=off  latency=0  precision=Full  arith_type=Unsigned  n_bits=16  bin_pt=14  quantization=Truncate  overflow=Wrap  dbl_ovrd=off  block_type=mux
  Dual Port RAM : xbsIndex_r4/Dual Port RAM  depth=1024  initVector=1:100  distributed_mem=Block RAM  init_a=0  init_b=0  rst_a=off  rst_b=off  en_a=off  en_b=off  latency=2  write_mode_A=Read After Write  write_mode_B=Read After Write  optimize=Speed  dbl_ovrd=off  block_type=dpram
  MA_addr : xbsIndex_r4/Slice  nbits=1  boolean_output=off  mode=Two Bit Locations  bit1=19  base1=LSB of Input  bit0=10  base0=LSB of Input  dbl_ovrd=off  block_type=slice
  MA_we : xbsIndex_r4/Slice  nbits=1  boolean_output=on  mode=Two Bit Locations  bit1=21  base1=LSB of Input  bit0=21  base0=LSB of Input  dbl_ovrd=off  block_type=slice
  MB_addr : xbsIndex_r4/Slice  nbits=1  boolean_output=off  mode=Two Bit Locations  bit1=9  base1=LSB of Input  bit0=0  base0=LSB of Input  dbl_ovrd=off  block_type=slice
  MB_we : xbsIndex_r4/Slice  nbits=1  boolean_output=on  mode=Two Bit Locations  bit1=20  base1=LSB of Input  bit0=20  base0=LSB of Input  dbl_ovrd=off  block_type=slice
  Mux2 : xbsIndex_r4/Mux  inputs=2  en=off  latency=0  precision=Full  arith_type=Unsigned  n_bits=16  bin_pt=14  quantization=Truncate  overflow=Wrap  dbl_ovrd=off  block_type=mux
  Mux9 : xbsIndex_r4/Mux  inputs=2  en=off  latency=0  precision=Full  arith_type=Unsigned  n_bits=16  bin_pt=14  quantization=Truncate  overflow=Wrap  dbl_ovrd=off  block_type=mux
  PA_sel : xbsIndex_r4/Slice  nbits=1  boolean_output=off  mode=Two Bit Locations  bit1=30  base1=LSB of Input  bit0=30  base0=LSB of Input  dbl_ovrd=off  block_type=slice
  Slice : xbsIndex_r4/Slice  nbits=1  boolean_output=off  mode=Two Bit Locations  bit1=16  base1=LSB of Input  bit0=9  base0=LSB of Input  dbl_ovrd=off  block_type=slice
  Slice1 : xbsIndex_r4/Slice  nbits=1  boolean_output=off  mode=Two Bit Locations  bit1=7  base1=LSB of Input  bit0=0  base0=LSB of Input  dbl_ovrd=off  block_type=slice
  Slice16 : xbsIndex_r4/Slice  nbits=1  boolean_output=off  mode=Two Bit Locations  bit1=16  base1=LSB of Input  bit0=16  base0=LSB of Input  dbl_ovrd=off  block_type=slice
  Slice18 : xbsIndex_r4/Slice  nbits=1  boolean_output=off  mode=Two Bit Locations  bit1=8  base1=LSB of Input  bit0=8  base0=LSB of Input  dbl_ovrd=off  block_type=slice
  Slice19 : xbsIndex_r4/Slice  nbits=1  boolean_output=off  mode=Two Bit Locations  bit1=8  base1=LSB of Input  bit0=8  base0=LSB of Input  dbl_ovrd=off  block_type=slice
  Slice2 : xbsIndex_r4/Slice  nbits=1  boolean_output=off  mode=Two Bit Locations  bit1=17  base1=LSB of Input  bit0=9  base0=LSB of Input  dbl_ovrd=off  block_type=slice
  Slice3 : xbsIndex_r4/Slice  nbits=1  boolean_output=off  mode=Two Bit Locations  bit1=8  base1=LSB of Input  bit0=0  base0=LSB of Input  dbl_ovrd=off  block_type=slice
  Slice4 : xbsIndex_r4/Slice  nbits=1  boolean_output=off  mode=Two Bit Locations  bit1=17  base1=LSB of Input  bit0=0  base0=LSB of Input  dbl_ovrd=off  block_type=slice
  Slice5 : xbsIndex_r4/Slice  nbits=1  boolean_output=off  mode=Two Bit Locations  bit1=35  base1=LSB of Input  bit0=18  base0=LSB of Input  dbl_ovrd=off  block_type=slice
  Slice6 : xbsIndex_r4/Slice  nbits=1  boolean_output=off  mode=Two Bit Locations  bit1=24  base1=LSB of Input  bit0=17  base0=LSB of Input  dbl_ovrd=off  block_type=slice
  Slice7 : xbsIndex_r4/Slice  nbits=1  boolean_output=off  mode=Two Bit Locations  bit1=24  base1=LSB of Input  bit0=17  base0=LSB of Input  dbl_ovrd=off  block_type=slice
  Slice8 : xbsIndex_r4/Slice  nbits=1  boolean_output=off  mode=Two Bit Locations  bit1=1  base1=LSB of Input  bit0=0  base0=LSB of Input  dbl_ovrd=off  block_type=slice
  X1 : xbsIndex_r4/AddSub  mode=Addition or Subtraction  use_carryin=off  use_carryout=off  en=off  latency=0  precision=User Defined  arith_type="Signed  (2's comp)"  n_bits=26  bin_pt=0  quantization=Truncate  overflow=Wrap  use_behavioral_HDL=off  hw_selection=Fabric  pipelined=off  dbl_ovrd=off  block_type=addsub
  X2 : xbsIndex_r4/AddSub  mode=Addition or Subtraction  use_carryin=off  use_carryout=off  en=off  latency=0  precision=User Defined  arith_type="Signed  (2's comp)"  n_bits=26  bin_pt=0  quantization=Truncate  overflow=Wrap  use_behavioral_HDL=off  hw_selection=Fabric  pipelined=off  dbl_ovrd=off  block_type=addsub
  bytemux : xbsIndex_r4/Mux  inputs=2  en=off  latency=0  precision=Full  arith_type=Unsigned  n_bits=16  bin_pt=14  quantization=Truncate  overflow=Wrap  dbl_ovrd=off  block_type=mux
  dn_ld : xbsIndex_r4/Slice  nbits=1  boolean_output=off  mode=Two Bit Locations  bit1=33  base1=LSB of Input  bit0=33  base0=LSB of Input  dbl_ovrd=off  block_type=slice
  sign : Subsystem
  up_ld : xbsIndex_r4/Slice  nbits=1  boolean_output=off  mode=Two Bit Locations  bit1=34  base1=LSB of Input  bit0=34  base0=LSB of Input  dbl_ovrd=off  block_type=slice
  w0 : xbsIndex_r4/Slice  nbits=1  boolean_output=off  mode=Two Bit Locations  bit1=8  base1=LSB of Input  bit0=0  base0=LSB of Input  dbl_ovrd=off  block_type=slice
  up_out : Outport
  down_out : Outport  Port=2
  Eout : Outport  Port=3
  wires:
  Convert4/1 -> "DSP48 Macro 3.0 "/1
  sign/2(sign1) -> Delay5/1
  w0/1 -> Bmux/5
  Convert10/1 -> "DSP48 Macro 3.0 "/3
  Dmux/1 -> Delay1/1
  Convert1/1 -> "DSP48 Macro 3.0 "/2
  Dual Port RAM/1 -> Delay10/1
  Slice2/1 -> bytemux/3
  Slice18/1 -> sign/2(signa1)
  Slice19/1 -> sign/3(signb)
  sign/1(sign0) -> Delay3/1
  PA_sel/1 -> BImux/1, AImux/1
  B_sel/1 -> Bmux/1
  Bbyte_sel/1 -> bytemux/1
  X1/1 -> Delay6/1
  MA_addr/1 -> Dual Port RAM/1
  MA_we/1 -> Dual Port RAM/3
  Slice5/1 -> AImux/3, X2/2
  Concat1/1 -> BImux/2
  Delay6/1 -> Slice7/1, X1/1
  Convert5/1 -> Slice5/1, Slice4/1
  X2/1 -> Delay4/1
  Acc_rst/1 -> Delay4/2, Delay6/2
  Delay4/1 -> Slice6/1, X2/1
  Slice4/1 -> BImux/3, X1/2
  Convert3/1 -> X1/3
  Constant1/1 -> Concat/2
  Slice6/1 -> Concat1/1
  "DSP48 Macro 3.0 "/1 -> Convert5/1
  Slice7/1 -> Concat1/2
  BImux/1 -> Delay7/1
  MB_we/1 -> Dual Port RAM/6
  Slice1/1 -> Concat/3
  Slice/1 -> Concat/1
  Slice3/1 -> bytemux/2
  Bmux/1 -> Delay2/1
  bytemux/1 -> Eout/1, Bmux/2
  Dual Port RAM/2 -> Delay11/1
  Weight_in/1 -> Dmux/3, w0/1
  Slice16/1 -> sign/1(signa0)
  Mux9/1 -> down_out/1
  dn_ld/1 -> Mux9/1
  D_sel/1 -> Dmux/1
  down_in/1 -> AImux/2, Dmux/4, Mux9/2
  Concat2/1 -> Convert2/1
  mode/1 -> Delay9/1
  up_in/1 -> Mux2/2, Dmux/5
  MB_addr/1 -> Dual Port RAM/4
  E_in/1 -> Bmux/3
  up_ld/1 -> Mux2/1
  Convert2/1 -> "DSP48 Macro 3.0 "/4
  Convert6/1 -> X2/3
  AImux/1 -> Delay8/1
  Mux2/1 -> up_out/1
  Delay1/1 -> Slice1/1, Slice18/1, Slice/1, Slice16/1
  Delay2/1 -> Slice19/1, Convert10/1
  Delay3/1 -> Convert6/1
  Delay5/1 -> Convert3/1
  Delay7/1 -> Dual Port RAM/5
  Delay8/1 -> Dual Port RAM/2
  Concat/1 -> Convert4/1
  Slice8/1 -> "DSP48 Macro 3.0 "/5
  DSP_op/1 -> Delay12/1
  Delay9/1 -> dn_ld/1, PA_sel/1, B_sel/1, MB_addr/1, MA_addr/1, MB_we/1, MA_we/1, DSP_op/1, Acc_rst/1, Bbyte_sel/1, D_sel/1, up_ld/1
  Delay10/1 -> Bmux/4, Convert1/1, Concat2/1
  Delay11/1 -> Slice3/1, Slice2/1, Concat2/2, Mux2/3, Mux9/3, Dmux/2
  Delay12/1 -> Slice8/1

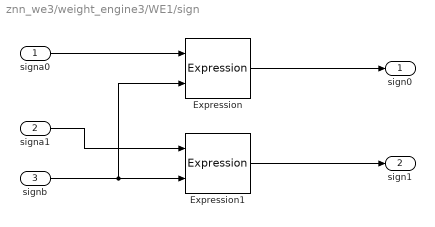
== system znn_we3/weight_engine3/WE1/sign ==
  signa0 : Inport
  signa1 : Inport  Port=2
  signb : Inport  Port=3
  Expression : xbsIndex_r4/Expression  expression=a ^ b  align_bp=on  en=off  latency=0  precision=Full  arith_type=Unsigned  n_bits=16  bin_pt=0  dbl_ovrd=off  block_type=expr
  Expression1 : xbsIndex_r4/Expression  expression=a ^ b  align_bp=on  en=off  latency=0  precision=Full  arith_type=Unsigned  n_bits=16  bin_pt=0  dbl_ovrd=off  block_type=expr
  sign0 : Outport
  sign1 : Outport  Port=2
  wires:
  signa0/1 -> Expression/1
  Expression/1 -> sign0/1
  signb/1 -> Expression1/2, Expression/2
  signa1/1 -> Expression1/1
  Expression1/1 -> sign1/1

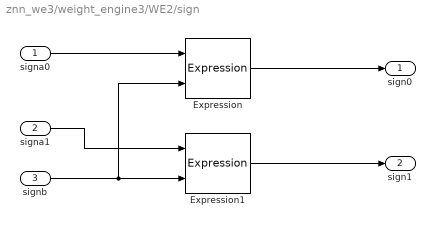
== system znn_we3/weight_engine3/WE2/sign ==
  signa0 : Inport
  signa1 : Inport  Port=2
  signb : Inport  Port=3
  Expression : xbsIndex_r4/Expression  expression=a ^ b  align_bp=on  en=off  latency=0  precision=Full  arith_type=Unsigned  n_bits=16  bin_pt=0  dbl_ovrd=off  block_type=expr
  Expression1 : xbsIndex_r4/Expression  expression=a ^ b  align_bp=on  en=off  latency=0  precision=Full  arith_type=Unsigned  n_bits=16  bin_pt=0  dbl_ovrd=off  block_type=expr
  sign0 : Outport
  sign1 : Outport  Port=2
  wires:
  signa0/1 -> Expression/1
  Expression/1 -> sign0/1
  signb/1 -> Expression1/2, Expression/2
  signa1/1 -> Expression1/1
  Expression1/1 -> sign1/1
